simulink subsystem "EE_Dyn"  (R2022a)
settings: Solver=VariableStepAuto  StartTime=0.0  StopTime=10.0  RelTol=1e-3
model mask{spaceRobot=sr, Xee0=0}
  mask prompts: Xee0 "EE Inital Position"
settings Model: Creator=charl  LastModifiedBy=charl

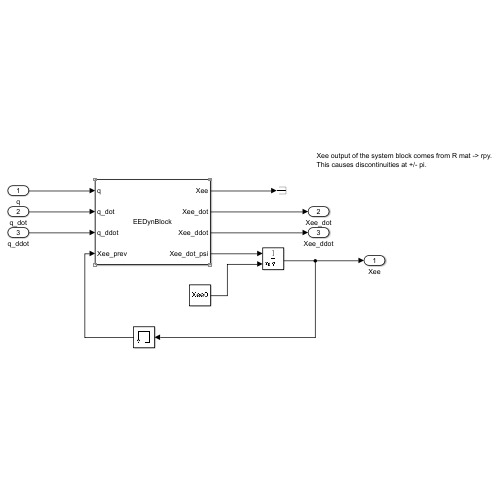
[thumbnail: Simulink's stored preview of the top-level diagram]
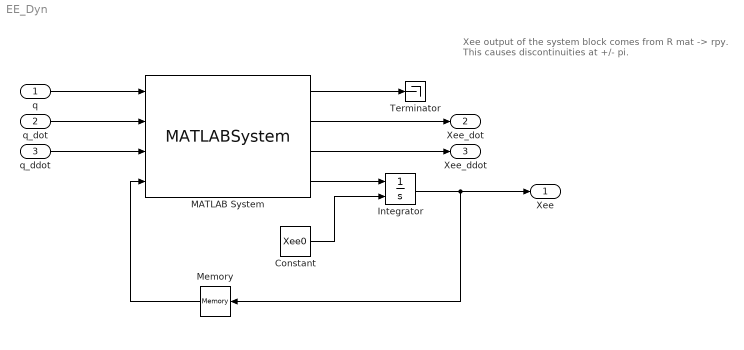
== system EE_Dyn ==
  note: Xee output of the system block comes from R mat -> rpy.
      | This causes discontinuities at +/- pi.
  q : Inport
  q_dot : Inport  Port=2
  q_ddot : Inport  Port=3
  Constant : Constant  Value=Xee0
  Integrator : Integrator  InitialConditionSource=external
  MATLAB System : MATLABSystem  System=EEDynBlock  srInfo=srInfo  srInfoFunc=srInfoFunc  srStateFunc=srStateFunc  srStateFuncMex=srStateFuncMex  SimulateUsing=Interpreted execution
      mask Type: EEDynBlock
      mask Display:
      | disp('EEDynBlock');
      | port_label('input',1,'q');
      | port_label('input',2,'q_dot');
      | port_label('input',3,'q_ddot');
      | port_label('input',4,'Xee_prev');
      | port_label('output',1,'Xee');
      | port_label('output',2,'Xee_dot');
      | port_label('output',3,'Xee_ddot');
      | port_label('output',4,'Xee_dot_psi');
  Memory : Memory
  Terminator : Terminator
  Xee : Outport
  Xee_dot : Outport  Port=2
  Xee_ddot : Outport  Port=3
  wires:
  q_dot/1 -> MATLAB System/2
  q/1 -> MATLAB System/1
  MATLAB System/1 -> Terminator/1
  MATLAB System/2 -> Xee_dot/1
  q_ddot/1 -> MATLAB System/3
  MATLAB System/3 -> Xee_ddot/1
  MATLAB System/4 -> Integrator/1
  Integrator/1 -> Xee/1, Memory/1
  Constant/1 -> Integrator/2
  Memory/1 -> MATLAB System/4
